simulink library "wt_blockset_v3"  (Simulink 6.0)
settings: Solver=ode45  SolverMode=SingleTasking  StartTime=0.0  StopTime=10.0  RelTol=1e-3
undefined symbols (not defined in the file): f1, get, j, Kmode, Type, u0
libraries: simulink_extras x12, simulink3 x5, simulink x4, dspinverses x1, dspmtrx3 x1, dspsnks4 x1
(part 2 of 7)

== system wt_blockset_v3/Electrical Machinery/Simulink Blocks  based Models ==
  note: Electric Machines Dynamic Models
  note: RMS Models
  note: Simulink Blocks
      |  based Models
  note: Special Models
  note: DQ Reference frame
  note: ABC/abc Models
  note: Salient Pole
      | Synchronous Machine
  note: Salient Pole
      | Synchronous Machine
  note: Reduced Order Models
  note: Permanent Magnet
      | Synchronous Machine
  note: Permanent Magnet
      | Synchronous Machine
  ABC/abc Squirell-Cage Induction Machine : Subsystem  mask(ABC/abc model of Squirrel Cage Induction Machine){Op_Mode=Generator, ConnType=Y, stator=[0.005 4.0744e-004], rotor=[0.0089 2.9921e-004], Lm=0.0160, p=2, init_cond=[0 0 0 0 0 0 0]}
      mask prompts: Op_Mode "Operating mode"; ConnType "Connection type"; stator "Stator windings [Rs Lsgm_s] [ohms H]"; rotor "Rotor windings [Rr Lsgm_r] [ohms H]"; Lm "Magnetizing inductance [H]"; p "Number of poles pair"; init_cond "Initial condition [iA iB iC ia ib ic theta]"
      mask help:
      | Implements an ABC/abc model for squirrel-cage induction machine.
      | Currents as state variable.
      mask init:
      | %%%%%%%%%%%%%%%%%%%%%%%%%%%%%%%%%%%%%%%%%%%%%%%%%%%%%%%%%%%%%%%%%%%%%%%%%%%%
      | % Matrix Coefficients for ABC/abc Model of Squirrel Cage Induction Machine %
      | %                       Last Update 10.05.20002                            %
      | %%%%%%%%%%%%%%%%%%%%%%%%%%%%%%%%%%%%%%%%%%%%%%%%%%%%%%%%%%%%%%%%%%%%%%%%%%%%
      | 
      | Rs=stator(1);
      | Lsgm_s=stator(2);
      | 
      | Rr=rotor(1);
      | Lsgm_r=rotor(2);
      | 
      | Msr=2*Lm/3;
      | 
      | %Self inductances
      | Ls=Lsgm_s+Lm;
      | Lr=Lsgm_r+Lm;
      | 
      | K1=Ls*Lr/(Msr^2);
      | 
      | K2=(K1-3/4)/(K1-9/4);
      | 
      | K3=-(3/4)/(K1-9/4);
      | 
      | K4=-(1/Msr)/(K1-9/4);
      | 
      | dlt=2*pi/3;
      | 
      | a11=K2*Rs/Ls;
      | a12=K3*Rs/Ls;
      | a13=3*Msr*sqrt(3)*K4/4;
      | a14=K4*Rr;
      | a15=Msr*(K2-K3)/Ls;
      | a16=K2/Ls;
      | a17=K3/Ls;
      | 
      | a31=K4*Rs;
      | a32=Msr*(K2-K3)/Lr;
      | a33=K2*Rr/Lr;
      | a34=K3*Rr/Lr;
      | a35=3*Msr*sqrt(3)*K4/4;
      | a36=K4;
      | if ConnType==1,Type=1;else Type=-1;end
      | if Op_Mode==1, Kmode=1;else Kmode=-1;end
      mask StyleString: popup(Motor|Generator),popup(Y|D),edit,edit,edit,edit,edit
      mask Display: disp('ABC/abc\nSC_IM')
  ABC/abc Wound Rotor Induction Machine : Subsystem  mask(ABC/abc model of Wound Rotor Induction Machine){stator=[0.005 4.0744e-004], rotor=[0.0089 2.9921e-004], Lm=0.0160, p=2, init_cond=[0 0 0 0 0 0 0]}
      mask prompts: stator "Stator windings [Rs Lsgm_s] [ohms H]"; rotor "Rotor windings [Rr Lsgm_r] [ohms H]"; Lm "Magnetizing inductance [H]"; p "Number of poles pair"; init_cond "Initial condition [iA iB iC ia ib ic theta]"
      mask help:
      | Implements an ABC/abc model for wound-rotor induction machine.
      | Currents as state variable.
      mask init:
      | %%%%%%%%%%%%%%%%%%%%%%%%%%%%%%%%%%%%%%%%%%%%%%%%%%%%%%%%%%%%%%%%%%%%%%%%%%%%
      | % Matrix Coefficients for ABC/abc Model of Wound Rotor Induction Machine %
      | %                       Last Update 10.05.20002                            %
      | %%%%%%%%%%%%%%%%%%%%%%%%%%%%%%%%%%%%%%%%%%%%%%%%%%%%%%%%%%%%%%%%%%%%%%%%%%%%
      | 
      | Rs=stator(1);
      | Lsgm_s=stator(2);
      | 
      | Rr=rotor(1);
      | Lsgm_r=rotor(2);
      | 
      | Msr=2*Lm/3;
      | 
      | %Self inductances
      | Ls=Lsgm_s+Lm;
      | Lr=Lsgm_r+Lm;
      | 
      | K1=Ls*Lr/(Msr^2);
      | 
      | K2=(K1-3/4)/(K1-9/4);
      | 
      | K3=-(3/4)/(K1-9/4);
      | 
      | K4=-(1/Msr)/(K1-9/4);
      | 
      | dlt=2*pi/3;
      | 
      | a11=K2*Rs/Ls;
      | a12=K3*Rs/Ls;
      | a13=3*Msr*sqrt(3)*K4/4;
      | a14=K4*Rr;
      | a15=Msr*(K2-K3)/Ls;
      | a16=K2/Ls;
      | a17=K3/Ls;
      | a18=K4;
      | 
      | a31=K4*Rs;
      | a32=Msr*(K2-K3)/Lr;
      | a33=K2*Rr/Lr;
      | a34=K3*Rr/Lr;
      | a35=3*Msr*sqrt(3)*K4/4;
      | a36=K4;
      | a37=K2/Lr;
      | a38=K3/Lr;
      mask Display: disp('ABC/abc\nWR_IM')
  Permanent Magnet Synchronous Machine with iron losses : Subsystem  mask{R=6.1, T=20, Ld=.043, Lq=.043, Ke=.165, p=2, s=Without iron losses}
      mask prompts: R "Rs [ohm] -stator resitance"; T "T [C] temperature of PMSM"; Ld "Ld [H] d-axis inductance"; Lq "Lq [H] - q-axis inductance"; Ke "Ke [Wb] - magnet flux"; p "p, pole pairs"; s "Iron Losses switch"
      mask init:
      | Rs=R*(1+.009*(T-20));
      mask StyleString: edit,edit,edit,edit,edit,edit,popup(With iron losses| Without iron losses)
      mask Display: disp('PM_SM')
  RMS Wound Rotor Induction Machine : Subsystem  mask(Complex Steady-State Induction Machine){rated_vi=[960 1310], rated_fp=[50 2], standstill=[8.8 79.5], stator=[0.005 4.074e-4], rotor=[0.0089 2.992e-4], Lm=16.0428e-3}
      mask prompts: rated_vi "Rated voltage / current per phase [Vph_r (V), Iph_r (A)]"; rated_fp "Base frequency,  Number of pole pairs [fs (Hz), p]"; standstill "Starting current,  Phase angle at standstill [Ist (pu), phi_st (deg)]"; stator "Stator parameters [Rs (ohms), Lsgm_s (H)]"; rotor "Rotor parameters [Rr (ohms), Lsgm_r (H)]"; Lm "Magnetizing inductance [H]"
      mask help:
      | Complex Steady-State Model of Induction Machine.
      | Deep-bar effect taken into account.
      mask init:
      | p=rated_fp(2); omg_synch=2*pi*rated_fp(1);
      | Xm=omg_synch*Lm;
      | Rs=stator(1); Xsgm_s= omg_synch*stator(2); Xs=Xsgm_s+Xm;
      | Rr=rotor(1); Xsgm_r=omg_synch*rotor(2); Xr=Xsgm_r+Xm;
      | sbd=Rr*sqrt((Rs^2+Xs^2)/((Xm^2-Xs*Xr)^2+(Rs*Xr)^2));
      | Rr_sc=(rated_vi(1)*sqrt(1/(1+(tan(standstill(2)*pi/180))^2))/standstill(1)/rated_vi(2)-Rs);
      | kr=Rr_sc/Rr;
      | kx=(tan(standstill(2)*pi/180)*(Rs+Rr_sc)-Xsgm_s)/Xsgm_r;
      mask Display: disp('Steady_State\nModel')
  RMS  Squirrel Cage Induction Machine : Subsystem  mask(Squirrel-Cage Induction Machine){rated_vi=[960 1310], rated_fp=[50 2], standstill=[8.8 79.5], stator=[0.005 0.128], rotor=[0.0089 0.094], Xm=5.04}
      mask prompts: rated_vi "Rated voltage / current per phase [Vph_r (V), Iph_r (A)]"; rated_fp "Base frequency,  Number of pole pairs [fs (Hz), p]"; standstill "Starting current,  Phase angle at standstill [Ist (pu), phi_st (deg)]"; stator "Stator parameters [Rs Xsgm_s]  [ohms]"; rotor "Rotor parameters [Rr Xsgm_r] [ohms]"; Xm "Magnetizing reactance [ohms]"
      mask help: Steady-State Model of Squirrel-cage Induction Machine
      mask init:
      | %%%%%%%%%%%%%%%%%%%%%%%%%%%%%%%%%%%%%%%%%%%%%%%%%%%%%%%%%%%%%%%%%%%%%%%%%%%%%%%%%%%%%
      | % Initialisation file for Squirrel-Cage Induction Machine with Deep Bar Effect      %
      | % RMS model
      | %                           Last Update 06.06.2002 by FI                             %
      | %%%%%%%%%%%%%%%%%%%%%%%%%%%%%%%%%%%%%%%%%%%%%%%%%%%%%%%%%%%%%%%%%%%%%%%%%%%%%%%%%%%%%
      | 
      | %base angular speed
      | omg_base=2*pi*rated_fp(1);
      | 
      | %%%%%%%%%%%%%%%%%%%%%%%%%%%%
      | %Stator winding
      | %%%%%%%%%%%%%%%%%%%%%%%%%%%%
      | 
      | %Stator resistance
      | Rs=stator(1);
      | 
      | %Stator leakage inductance
      | Xsgm_s= stator(2);
      | 
      | %Stator self-inductance
      | Xs=Xsgm_s+Xm;
      | 
      | %%%%%%%%%%%%%%%%%%%%%%%%%%%%
      | %Rotor winding
      | %%%%%%%%%%%%%%%%%%%%%%%%%%%%
      | 
      | %Rotor resistance for rated operating point
      | Rr=rotor(1); 
      | 
      | %Rotor leakage inductance for rated operating point
      | Xsgm_r=rotor(2);
      | 
      | %Rotor self-inductance
      | Xr=Xsgm_r+Xm;
      | 
      | %Number of pole pairs
      | p=rated_fp(2);
      | 
      | %Breakdown slip
      | sbd=Rr*sqrt((Rs^2+Xs^2)/((Xm^2-Xs*Xr)^2+(Rs*Xr)^2));
      | 
      | %rotor resistance at start_up
      | Rr_sc=(rated_vi(1)*sqrt(1/(1+(tan(standstill(2)*pi/180))^2))/standstill(1)/rated_vi(2)-Rs);
      | 
      | %rotor resistance displacement factor
      | kr=Rr_sc/Rr;
      | 
      | %rotor reactance displacement factor
      | kx=(tan(standstill(2)*pi/180)*(Rs+Rr_sc)-Xsgm_s)/Xsgm_r;
      mask Display: disp('Steady_State\nModel')
  Reduced Order Model Induction Machine : Subsystem  mask(Generalized 3rd order model of Asynchronous Generator){stator=[0.0011, 7e-005], rotor=[0.0013, 7.5e-005], magnetization=2.9936e-003, rated_fp=[50 2], init_cond=[0 0]}
      mask prompts: stator "Stator parameters [Rs (ohms), Lsgm_s (H)]"; rotor "Rotor parameters [Rr (ohms), Lsgm_r (H)]"; magnetization "Magnetizing inductance Lm (H)"; rated_fp "Base frequency, Number of pole pairs [fs (Hz), p]"; init_cond "Initial conditions [fi_dr (Wb), fi_qr(Wb)]"
      mask help: Implements a generalized 3rd order model for Asynchronous Generator in synchronous reference frame.
      mask init:
      | Rs=stator(1);Lsgm_s=stator(2);
      | Rr=rotor(1);Lsgm_r=rotor(2);Lm=magnetization;
      | omg_e=2*pi*rated_fp(1);p=rated_fp(2);
      | Lss=Lsgm_s+Lm;Lrr=Lsgm_r+Lm;D=Lss*Lrr-Lm^2;
      | tau_sr=Rs*Lrr/D;tau_rm=Rr*Lm/D;sigma_r=Lm/Lrr;sigma_s=Lm/Lss;
      | alpha=1/(1+(omg_e/tau_sr)^2);
      | M=[Lss 0 Lm 0;0 Lss 0 Lm;Lm 0 Lrr 0;0 Lm 0 Lrr];
      | Q=inv(M);
      mask Display: disp('IM\n3rd Order Model')
  Salient-Pole Synchronous Machine constant parameters : Subsystem  mask{stator_winding=[2.34e-3 3.92e-4], field_winding=[5e-4 6.69246e-4], rotor_winding=[17.36e-3 5.22558e-4 16.75e-3 3.36082e-4], mag_ind=[2.3844e-3 1.1759e-3], p=32}
      mask prompts: stator_winding "Stator winding [Rs Lsgm_s]"; field_winding "Field winding [Rf Lsgm_f]"; rotor_winding "Rotor winding [Rrd Lsgm_rd Rrq Lsgm_rq]"; mag_ind "Magnetizing inductances [Lmd Lmq]"; p "Number of pole pairs"
      mask init:
      | %%%%%%%%%%%%%%%%%%%%%%%%%%%%%%%%%%%%%%%%%%%%%%%%%%%%%%%%%%%%%%%%%%%%%%%%
      | % Matrix coefficients for DQ model of Salient-Pole Synchronous Machine %
      | %                   Last Update 10.05.2002                             %
      | %%%%%%%%%%%%%%%%%%%%%%%%%%%%%%%%%%%%%%%%%%%%%%%%%%%%%%%%%%%%%%%%%%%%%%%%
      | 
      | %Stator winding
      | Rs=stator_winding(1); Lsgm_s=stator_winding(2);
      | 
      | %Field winding
      | Rf=field_winding(1); Lsgm_f=field_winding(2);
      | 
      | %Rotor winding D axis
      | Rrd=rotor_winding(1); Lsgm_rd=rotor_winding(2);
      | 
      | %Rotor windin Q axis
      | Rrq=rotor_winding(3); Lsgm_rq=rotor_winding(4);
      | 
      | %Magnetizing inductances DQ axis
      | Lmd=mag_ind(1); Lmq=mag_ind(2);
      | 
      | %Self Inductances
      | Lssd=Lsgm_s+Lmd;
      | Lssq=Lsgm_s+Lmq;
      | Lsf=Lsgm_f+Lmd;
      | Lsrd=Lsgm_rd+Lmd;
      | Lsrq=Lsgm_rq+Lmq;
      | 
      | %Coeffients
      | Ksgm_d=Lsgm_s*Lsgm_f*Lsgm_rd+Lmd*(Lsgm_s*Lsgm_f+Lsgm_f*Lsgm_rd+Lsgm_rd*Lsgm_s);
      | Ksgm_q=Lsgm_s*Lsgm_rq+Lmq*(Lsgm_s+Lsgm_rq);
      | 
      | Ksgm_frd=Lsgm_f*Lsgm_rd+Lmd*(Lsgm_f+Lsgm_rd);
      | Ksgm_srd=Lsgm_s*Lsgm_rd+Lmd*(Lsgm_s+Lsgm_rd);
      | Ksgm_sf=Lsgm_f*Lsgm_s+Lmd*(Lsgm_f+Lsgm_s);
      | 
      | %Matrix coefficients
      | a11=-Rs*Ksgm_frd/Ksgm_d;
      | a12=Lssq*Ksgm_frd/Ksgm_d;
      | a13=Rf*Lsgm_rd*Lmd/Ksgm_d;
      | a14=Rrd*Lsgm_f*Lmd/Ksgm_d;
      | a15=Lmq*Ksgm_frd/Ksgm_d;
      | a16=Ksgm_frd/Ksgm_d;
      | a17=-Lsgm_rd*Lmd/Ksgm_d;
      | 
      | a21=-Lssd*Lsrq/Ksgm_q;
      | a22=-Rs*Lsrq/Ksgm_q;
      | a23=-Lsrq*Lmd/Ksgm_q;
      | a24=-Lsrq*Lmd/Ksgm_q;
      | a25=Rrq*Lmq/Ksgm_q;
      | a26=Lsrq/Ksgm_q;
      | 
      | a31=+Rs*Lsgm_rd*Lmd/Ksgm_d;
      | a32=-Lssq*Lsgm_rd*Lmd/Ksgm_d;
      | a33=-Rf*Ksgm_srd/Ksgm_d;
      | a34=Rrd*Lsgm_s*Lmd/Ksgm_d;
      | a35=-Lsgm_rd*Lmd*Lmq/Ksgm_d;
      | a36=-Lsgm_rd*Lmd/Ksgm_d;
      | a37=Ksgm_srd/Ksgm_d;
      | 
      | a41=Rs*Lsgm_f*Lmd/Ksgm_d;
      | a42=-Lsgm_f*Lssq*Lmd/Ksgm_d;
      | a43=Rf*Lsgm_s*Lmd/Ksgm_d;
      | a44=-Rrd*Ksgm_sf/Ksgm_d;
      | a45=-Lsgm_f*Lmd*Lmq/Ksgm_d;
      | a46=-Lsgm_f*Lmd/Ksgm_d;
      | a47=-Lsgm_s*Lmd/Ksgm_d;
      | 
      | a51=Lssd*Lmq/Ksgm_q;
      | a52=Rs*Lmq/Ksgm_q;
      | a53=Lmd*Lmq/Ksgm_q;
      | a54=Lmd*Lmq/Ksgm_q;
      | a55=-Rrq*Lssq/Ksgm_q;
      | a56=-Lmq/Ksgm_q;
      mask Display: disp('SP_SM')
  Squirrel Cage Induction Machine constant parameters : Subsystem  mask(Squirrel-Cage Induction Machine){Op_Mode=Generator, ConnType=Y, stator=[3.67 9.2e-3], rotor=[2.32 12.29e-3], Lm=0.235, p=2, x0=[0 0 0 0 0]}
      mask prompts: Op_Mode "Operating mode"; ConnType "Connection type"; stator "Stator parameters [Rs (ohm), Lsgm_s(H)]"; rotor "Rotor parameters [Rr (ohm) Lsgm_r (H)]"; Lm "Mutual inductance [H]"; p "Number of pole pairs"; x0 "Initial conditions [ids iqs idr iqr theta]"
      mask help:
      | Implements a dq model in rotor reference frame for squirrel-cage induction machine.
      | Currents as state variable.
      mask init:
      | if ConnType==1,Type=1;else Type=-1;end
      | if Op_Mode==1, Kmode=1;else Kmode=-1;end
      | Rs=stator(1); Lsgms= stator(2); Lss=Lsgms+Lm;
      | Rr=rotor(1); Lsgmr=rotor(2); Lsr=Lsgmr+Lm;
      | sigma=1-(Lm*Lm)/(Lss*Lsr);
      mask StyleString: popup(Motor|Generator),popup(Y|D),edit,edit,edit,edit,edit
      mask Display: disp('SC_IM')
  Squirrel Cage  Induction Machine  with Deep Bar Effect : Subsystem  mask(Squirrel-Cage Induction Machine with Deep Bar Effect){Op_Mode=Motor, ConnType=Y, rated_vi=[960 1310], rated_fp=[50 2], standstill=[8.8 79.5], stator=[0.005 4.074e-4], rotor=[0.0089 2.992e-4], Lm=16.0428e-3, x0=[0 0 0 0 0]}
      mask prompts: Op_Mode "Operating mode"; ConnType "Connection type"; rated_vi "Rated voltage / current per-phase [Vph_r (V), Iph_r (A)]"; rated_fp "Base frequency,  Number of pole pairs [fs (Hz), p]"; standstill "Starting current,  Phase angle at standstill [Ist (pu), phi_st (deg)]"; stator "Stator [Rs (ohm), Lsgm_s (H)]"; rotor "Rotor [Rr (ohm), Lsgm_r (H)]"; Lm "Magnetizing inductance Lm [H]"; x0 "Initial conditions [ids iqs idr iqr theta]"
      mask help: Implement a DQ Model in rotor reference frame for Squirrel-Cage Induction Machine with Deep bar effect
      mask init:
      | if ConnType==1,Type=1;else Type=-1;end
      | if Op_Mode==1, Kmode=1;else Kmode=-1;end
      | %%%%%%%%%%%%%%%%%%%%%%%%%%%%%%%%%%%%%%%%%%%%%%%%%%%%%%%%%%%%%%%%%%%%%%%%%%%%%%%%%%%%%
      | % Initialisation file for squirrel-Cage Induction Machine with Deep Bar Effect      %
      | %                          Last Update 15.05.2002 by FI                             %
      | %%%%%%%%%%%%%%%%%%%%%%%%%%%%%%%%%%%%%%%%%%%%%%%%%%%%%%%%%%%%%%%%%%%%%%%%%%%%%%%%%%%%%
      | 
      | %base angular speed
      | omg_base=2*pi*rated_fp(1);
      | 
      | %Magnetizing reactance
      | Xm=omg_base*Lm;
      | %%%%%%%%%%%%%%%%%%%%%%%%%%%%
      | %Stator winding
      | %%%%%%%%%%%%%%%%%%%%%%%%%%%%
      | 
      | %Stator resistance
      | Rs=stator(1);
      | 
      | %Stator leakage inductance
      | Lsgms= stator(2);
      | Xsgm_s=omg_base*Lsgms;
      | 
      | %Stator self-inductance
      | Lss=Lsgms+Lm;
      | Xs=omg_base*Lss;
      | 
      | %%%%%%%%%%%%%%%%%%%%%%%%%%%%
      | %Rotor winding
      | %%%%%%%%%%%%%%%%%%%%%%%%%%%%
      | 
      | %Rotor resistance for rated operating point
      | Rr=rotor(1); 
      | 
      | %Rotor leakage inductance for rated operating point
      | Lsgmr=rotor(2);
      | Xsgm_r=omg_base*rotor(2);
      | 
      | %Rotor self-inductance
      | Lsr=rotor(2)+Lm;
      | Xr=omg_base*Lsr;
      | 
      | %Number of pole pairs
      | p=rated_fp(2);
      | 
      | %Breakdown slip
      | sbd=Rr*sqrt((Rs^2+Xs^2)/((Xm^2-Xs*Xr)^2+(Rs*Xr)^2));
      | 
      | %rotor resistance at start_up
      | Rr_sc=(rated_vi(1)*sqrt(1/(1+(tan(standstill(2)*pi/180))^2))/standstill(1)/rated_vi(2)-Rs);
      | 
      | %rotor resistance displacement factor
      | kr=Rr_sc/Rr;
      | 
      | %rotor reactance displacement factor
      | kx=(tan(standstill(2)*pi/180)*(Rs+Rr_sc)-Xsgm_s)/Xsgm_r;
      mask StyleString: popup(Motor|Generator),popup(Y|D),edit,edit,edit,edit,edit,edit,edit
      mask Display: disp('SC_IM')
  Wound Rotor Induction Machine constant parameters : Subsystem  mask(3-phase Wound Rotor Induction Machine){stator=[0.01 95.5e-6], rotor=[0.01 95.5e-6], Lm=0.0955, p=2, x0=[0 0 0 0 0]}
      mask prompts: stator "Stator parameters [Rs (ohm), Lsgm_s (H)]"; rotor "Rotor parameters [Rr (ohm), Lsgm_r (H)]"; Lm "Magnetizing inductance [H]"; p "Number of poles pair"; x0 "Initial conditions [ids iqs idr' iqr' theta]"
      mask init:
      | Rs=stator(1); Lsgm_s=stator(2);
      | Rr=rotor(1); Lsgm_r=rotor(2);
      | Lss=Lsgm_s+Lm;
      | Lsr=Lsgm_r+Lm;
      | sigma=1-(Lm*Lm)/(Lss*Lsr);
      mask Display: disp('WR_IM')
  "Wound Rotor Induction Machine with Deep Bar Effect " : Subsystem  mask(3-phase Wound Rotor Induction Machine){rated_vi=[960 1310], rated_fp=[50 2], standstill=[8.8 79.5], stator=[0.005 4.074e-4], rotor=[0.0089 2.992e-4], Lm=16.0428e-3, x0=[0 0 0 0 0]}
      mask prompts: rated_vi "Rated voltage / current per-phase [Vph_r (V), Iph_r (A)]"; rated_fp "Base frequency,  Number of pole pairs [fs (Hz), p]"; standstill "Starting current,  Phase angle at standstill [Ist (pu), phi_st (deg)]"; stator "Stator [Rs (ohm), Lsgm_s (H)]"; rotor "Rotor [Rr (ohm), Lsgm_r (H)]"; Lm "Magnetizing inductance Lm [H]"; x0 "Initial conditions [ids iqs idr' iqr' theta]"
      mask init:
      | %%%%%%%%%%%%%%%%%%%%%%%%%%%%%%%%%%%%%%%%%%%%%%%%%%%%%%%%%%%%%%%%%%%%%%%%%%%%%%%%%%%%%
      | % Initialisation file for Wound Rotor Induction Machine with Deep Bar Effect      %
      | %                          Last Update 24.09.2004 by FI                             %
      | %%%%%%%%%%%%%%%%%%%%%%%%%%%%%%%%%%%%%%%%%%%%%%%%%%%%%%%%%%%%%%%%%%%%%%%%%%%%%%%%%%%%%
      | 
      | %base angular speed
      | omg_base=2*pi*rated_fp(1);
      | 
      | %Magnetizing reactance
      | Xm=omg_base*Lm;
      | %%%%%%%%%%%%%%%%%%%%%%%%%%%%
      | %Stator winding
      | %%%%%%%%%%%%%%%%%%%%%%%%%%%%
      | 
      | %Stator resistance
      | Rs=stator(1);
      | 
      | %Stator leakage inductance
      | Lsgms= stator(2);
      | Xsgm_s=omg_base*Lsgms;
      | 
      | %Stator self-inductance
      | Lss=Lsgms+Lm;
      | Xs=omg_base*Lss;
      | 
      | %%%%%%%%%%%%%%%%%%%%%%%%%%%%
      | %Rotor winding
      | %%%%%%%%%%%%%%%%%%%%%%%%%%%%
      | 
      | %Rotor resistance for rated operating point
      | Rr=rotor(1); 
      | 
      | %Rotor leakage inductance for rated operating point
      | Lsgmr=rotor(2);
      | Xsgm_r=omg_base*rotor(2);
      | 
      | %Rotor self-inductance
      | Lsr=rotor(2)+Lm;
      | Xr=omg_base*Lsr;
      | 
      | %Number of pole pairs
      | p=rated_fp(2);
      | 
      | %Breakdown slip
      | sbd=Rr*sqrt((Rs^2+Xs^2)/((Xm^2-Xs*Xr)^2+(Rs*Xr)^2));
      | 
      | %rotor resistance at start_up
      | Rr_sc=(rated_vi(1)*sqrt(1/(1+(tan(standstill(2)*pi/180))^2))/standstill(1)/rated_vi(2)-Rs);
      | 
      | %rotor resistance displacement factor
      | kr=Rr_sc/Rr;
      | 
      | %rotor reactance displacement factor
      | kx=(tan(standstill(2)*pi/180)*(Rs+Rr_sc)-Xsgm_s)/Xsgm_r;
      mask Display: disp('WR_IM')

== system wt_blockset_v3/Grid Models/3-ph line 1 ==
  note: VfR
  note: VbR
  note: VfS
  note: VbS
  iS_abc : Inport  Port=1  LatchInput=off
  iR_abc : Inport  Orientation=left  Port=2  LatchInput=off
  1 : Gain  Gain=atten  SaturateOnIntegerOverflow=on
  2 : Gain  Orientation=left  Gain=atten  SaturateOnIntegerOverflow=on
  Gain1 : Gain  Orientation=left  Gain=2  SaturateOnIntegerOverflow=on
  Gain6 : Gain  Gain=2  SaturateOnIntegerOverflow=on
  R_to_S delay : TransportDelay  Orientation=left  DelayTime=tdelay  BufferSize=buffer_size
  S_to_R delay : TransportDelay  DelayTime=tdelay  BufferSize=buffer_size
  Sum1 : Sum  Orientation=up  SaturateOnIntegerOverflow=on  InputSameDT=on
  Sum2 : Sum  Inputs=+-  SaturateOnIntegerOverflow=on  InputSameDT=on
  Sum4 : Sum  Orientation=down  Inputs=+-  SaturateOnIntegerOverflow=on  InputSameDT=on
  Sum5 : Sum  Orientation=left  Inputs=-+  SaturateOnIntegerOverflow=on  InputSameDT=on
  Zc1 : Gain  Orientation=up  Gain=Zc  SaturateOnIntegerOverflow=on
  Zc2 : Gain  Orientation=down  Gain=Zc  SaturateOnIntegerOverflow=on
  VS_abc : Outport  Orientation=left  InitialOutput=0
  "VR_abc " : Outport  Port=2  InitialOutput=0
  wires:
  1/1 -> Sum5/1, Gain6/1
  Sum1/1 -> Sum2/1, VS_abc/1
  iR_abc/1 -> Zc2/1
  iS_abc/1 -> Zc1/1
  Sum4/1 -> "VR_abc "/1, Sum5/2
  Sum5/1 -> R_to_S delay/1
  Zc2/1 -> Sum4/2
  Sum2/1 -> S_to_R delay/1
  Zc1/1 -> Sum1/1
  Gain6/1 -> Sum4/1
  Gain1/1 -> Sum1/2
  S_to_R delay/1 -> 1/1
  R_to_S delay/1 -> 2/1
  2/1 -> Gain1/1, Sum2/2

== system wt_blockset_v3/Grid Models/3-ph line 2 ==
  note: VbS
  note: VfS
  note: VbR
  note: VfR
  VS_abc : Inport  Port=1  LatchInput=off
  iR_abc : Inport  Orientation=left  Port=2  LatchInput=off
  3 : Gain  Gain=atten  SaturateOnIntegerOverflow=on
  4 : Gain  Orientation=left  Gain=atten  SaturateOnIntegerOverflow=on
  Gain3 : Gain  Gain=2  SaturateOnIntegerOverflow=on
  Gain4 : Gain  Orientation=left  Gain=2  SaturateOnIntegerOverflow=on
  R_to_S delay1 : TransportDelay  Orientation=left  DelayTime=tdelay  BufferSize=buffer_size
  S_to_R delay1 : TransportDelay  DelayTime=tdelay  BufferSize=buffer_size
  Sum2 : Sum  Inputs=+-  SaturateOnIntegerOverflow=on  InputSameDT=on
  Sum3 : Sum  Inputs=+-  SaturateOnIntegerOverflow=on  InputSameDT=on
  Sum6 : Sum  Orientation=down  Inputs=+-  SaturateOnIntegerOverflow=on  InputSameDT=on
  Sum7 : Sum  Orientation=left  Inputs=-+  SaturateOnIntegerOverflow=on  InputSameDT=on
  Zc3 : Gain  Gain=1/Zc  SaturateOnIntegerOverflow=on
  Zc4 : Gain  Orientation=down  Gain=Zc  SaturateOnIntegerOverflow=on
  break algebraic loop1 : Subsystem  mask(Transfer function){K=1, T=1e-5, x0=445}
      mask prompts: K "Gain"; T "Time constant"; x0 "Initial condition"
      mask help: Implements a transfer function K/(sT+1) with initial condition.
  iS_abc : Outport  InitialOutput=0
  "VR_abc " : Outport  Port=2  InitialOutput=0
  wires:
  4/1 -> Sum3/2, Gain4/1
  R_to_S delay1/1 -> 4/1
  S_to_R delay1/1 -> 3/1
  Gain3/1 -> Sum6/1
  Sum3/1 -> S_to_R delay1/1
  Zc4/1 -> Sum6/2
  Sum7/1 -> R_to_S delay1/1
  Sum6/1 -> Sum7/2, "VR_abc "/1
  3/1 -> Sum7/1, Gain3/1
  VS_abc/1 -> Sum2/1, Sum3/1
  iR_abc/1 -> Zc4/1
  Zc3/1 -> break algebraic loop1/1(In1)
  Sum2/1 -> Zc3/1
  Gain4/1 -> Sum2/2
  break algebraic loop1/1(Out1) -> iS_abc/1

== system wt_blockset_v3/Grid Models/3-phase 3 limb  C S-Function ==
  v_UVW : Inport  Port=1  LatchInput=off
  i_uvw : Inport  Port=2  LatchInput=off
  Mux : Mux  Inputs=2
  Ropen : Gain  Orientation=down  Gain=1000000  SaturateOnIntegerOverflow=on
  Ropen1 : Gain  Gain=-sqrt(3)  SaturateOnIntegerOverflow=on
  S-Function : S-Function  FunctionName=trafo3limb_abc_zcs  Parameters=a b init_cond
  Selector iABC : Selector  Elements=[1 2 3]  InputPortWidth=6
  Selector iabc : Selector  Elements=[4 5 6]  InputPortWidth=6
  Sum : Sum  Inputs=|+-  SaturateOnIntegerOverflow=on  InputSameDT=on
  phase->line2 : Subsystem
  turns ratio : Gain  Gain=-alpha_T  SaturateOnIntegerOverflow=on
  turns ratio1 : Gain  Gain=alpha_T  SaturateOnIntegerOverflow=on
  i_UVW : Outport
  v_uvw : Outport  Port=2
  wires:
  i_uvw/1 -> Sum/2
  turns ratio1/1 -> Sum/1
  Ropen1/1 -> v_uvw/1
  Ropen/1 -> turns ratio/1, Ropen1/1
  Sum/1 -> Ropen/1
  S-Function/1 -> Selector iabc/1, Selector iABC/1
  Mux/1 -> S-Function/1
  turns ratio/1 -> Mux/2
  v_UVW/1 -> Mux/1
  phase->line2/1(out) -> i_UVW/1
  Selector iABC/1 -> phase->line2/1(in)
  Selector iabc/1 -> turns ratio1/1

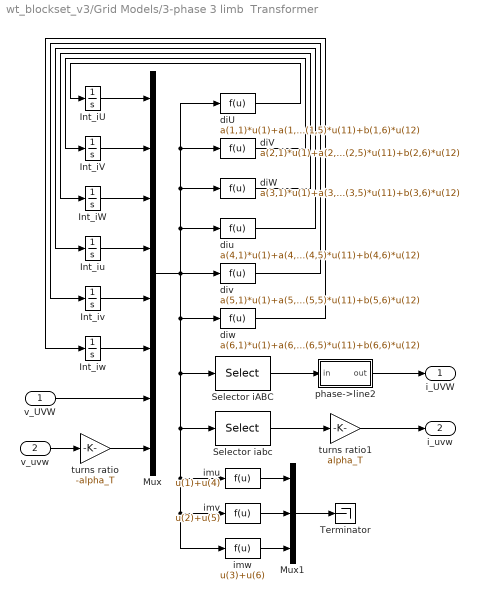
== system wt_blockset_v3/Grid Models/3-phase 3 limb  Transformer ==
  v_UVW : Inport  Port=1  LatchInput=off
  v_uvw : Inport  Port=2  LatchInput=off
  Int_iU : Integrator
  Int_iV : Integrator
  Int_iW : Integrator
  Int_iu : Integrator
  Int_iv : Integrator
  Int_iw : Integrator
  Mux : Mux  Inputs=[1 1 1 1 1 1 3 3]
  Mux1 : Mux  Inputs=3
  Selector iABC : Selector  Elements=[1 2 3]  InputPortWidth=12
  Selector iabc : Selector  Elements=[4 5 6]  InputPortWidth=12
  Terminator : Terminator
  diU : Fcn  Expr=a(1,1)*u(1)+a(1,2)*u(2)+a(1,3)*u(3)+a(1,4)*u(4)+a(1,5)*u(5)+a(1,6)*u(6)+b(1,1)*u(7)+b(1,2)*u(8)+b(1,3)*u(9)+b(1,4)*u(10)+b(1,5)*u(11)+b(1,6)*u(12)
  diV : Fcn  Expr=a(2,1)*u(1)+a(2,2)*u(2)+a(2,3)*u(3)+a(2,4)*u(4)+a(2,5)*u(5)+a(2,6)*u(6)+b(2,1)*u(7)+b(2,2)*u(8)+b(2,3)*u(9)+b(2,4)*u(10)+b(2,5)*u(11)+b(2,6)*u(12)
  diW : Fcn  Expr=a(3,1)*u(1)+a(3,2)*u(2)+a(3,3)*u(3)+a(3,4)*u(4)+a(3,5)*u(5)+a(3,6)*u(6)+b(3,1)*u(7)+b(3,2)*u(8)+b(3,3)*u(9)+b(3,4)*u(10)+b(3,5)*u(11)+b(3,6)*u(12)
  diu : Fcn  Expr=a(4,1)*u(1)+a(4,2)*u(2)+a(4,3)*u(3)+a(4,4)*u(4)+a(4,5)*u(5)+a(4,6)*u(6)+b(4,1)*u(7)+b(4,2)*u(8)+b(4,3)*u(9)+b(4,4)*u(10)+b(4,5)*u(11)+b(4,6)*u(12)
  div : Fcn  Expr=a(5,1)*u(1)+a(5,2)*u(2)+a(5,3)*u(3)+a(5,4)*u(4)+a(5,5)*u(5)+a(5,6)*u(6)+b(5,1)*u(7)+b(5,2)*u(8)+b(5,3)*u(9)+b(5,4)*u(10)+b(5,5)*u(11)+b(5,6)*u(12)
  diw : Fcn  Expr=a(6,1)*u(1)+a(6,2)*u(2)+a(6,3)*u(3)+a(6,4)*u(4)+a(6,5)*u(5)+a(6,6)*u(6)+b(6,1)*u(7)+b(6,2)*u(8)+b(6,3)*u(9)+b(6,4)*u(10)+b(6,5)*u(11)+b(6,6)*u(12)
  imu : Fcn  Expr=u(1)+u(4)
  imv : Fcn  Expr=u(2)+u(5)
  imw : Fcn  Expr=u(3)+u(6)
  phase->line2 : Subsystem
  turns ratio : Gain  Gain=-alpha_T  SaturateOnIntegerOverflow=on
  turns ratio1 : Gain  Gain=alpha_T  SaturateOnIntegerOverflow=on
  i_UVW : Outport
  i_uvw : Outport  Port=2
  wires:
  turns ratio/1 -> Mux/8
  Selector iabc/1 -> turns ratio1/1
  Selector iABC/1 -> phase->line2/1(in)
  v_uvw/1 -> turns ratio/1
  v_UVW/1 -> Mux/7
  diw/1 -> Int_iw/1
  div/1 -> Int_iv/1
  diu/1 -> Int_iu/1
  diW/1 -> Int_iW/1
  diV/1 -> Int_iV/1
  diU/1 -> Int_iU/1
  Int_iw/1 -> Mux/6
  Int_iv/1 -> Mux/5
  Int_iu/1 -> Mux/4
  Int_iW/1 -> Mux/3
  Int_iV/1 -> Mux/2
  Int_iU/1 -> Mux/1
  Mux/1 -> Selector iABC/1, Selector iabc/1, imu/1, imv/1, imw/1, diw/1, div/1, diU/1, diV/1, diW/1, diu/1
  turns ratio1/1 -> i_uvw/1
  phase->line2/1(out) -> i_UVW/1
  imu/1 -> Mux1/1
  imv/1 -> Mux1/2
  imw/1 -> Mux1/3
  Mux1/1 -> Terminator/1

== system wt_blockset_v3/Grid Models/3-phase source ==
  Mux3 : Mux  Inputs=3
  ua : Sin  Amplitude=sqrt(2)*Uf  Frequency=2*pi*fs  SampleTime=0
  ub : Sin  Amplitude=sqrt(2)*Uf  Frequency=2*pi*fs  Phase=-2*pi/3  SampleTime=0
  uc : Sin  Amplitude=sqrt(2)*Uf  Frequency=2*pi*fs  Phase=2*pi/3  SampleTime=0
  uRST : Outport  InitialOutput=0
  wires:
  uc/1 -> Mux3/3
  ub/1 -> Mux3/2
  Mux3/1 -> uRST/1
  ua/1 -> Mux3/1

== system wt_blockset_v3/Grid Models/Capacitor Bank RC ==
  V_RST : Inport  Port=1  LatchInput=off
  k : Inport  Port=2  LatchInput=off
  Branch A : TransferFcn  Numerator=[C 0]  Denominator=[R*C 1]
  Branch B : TransferFcn  Numerator=[C 0]  Denominator=[R*C 1]
  Branch C : TransferFcn  Numerator=[C 0]  Denominator=[R*C 1]
  Demux : Demux  Outputs=3
  Mux : Mux  Inputs=3
  Product : Product  SaturateOnIntegerOverflow=on  InputSameDT=on
  I_RST : Outport
  wires:
  k/1 -> Product/2
  Product/1 -> I_RST/1
  V_RST/1 -> Demux/1
  Mux/1 -> Product/1
  Branch C/1 -> Mux/3
  Branch B/1 -> Mux/2
  Branch A/1 -> Mux/1
  Demux/3 -> Branch C/1
  Demux/2 -> Branch B/1
  Demux/1 -> Branch A/1

== system wt_blockset_v3/Grid Models/Capacitor Bank RC modified ==
  V_RST : Inport  Port=1  LatchInput=off
  k : Inport  Port=2  LatchInput=off
  Branch A : TransferFcn  Numerator=[C 0]  Denominator=[R*C 1]
  Branch B : TransferFcn  Numerator=[C 0]  Denominator=[R*C 1]
  Branch C : TransferFcn  Numerator=[C 0]  Denominator=[R*C 1]
  Demux : Demux  Outputs=3
  Mux : Mux  Inputs=3
  Product : Product  SaturateOnIntegerOverflow=on  InputSameDT=on
  I_RST : Outport
  wires:
  k/1 -> Product/2
  Product/1 -> I_RST/1
  V_RST/1 -> Demux/1
  Mux/1 -> Product/1
  Branch C/1 -> Mux/3
  Branch B/1 -> Mux/2
  Branch A/1 -> Mux/1
  Demux/3 -> Branch C/1
  Demux/2 -> Branch B/1
  Demux/1 -> Branch A/1

== system wt_blockset_v3/Grid Models/Capacitor Bank RLC ==
  v_RST : Inport  Port=1  LatchInput=off
  k : Inport  Port=2  LatchInput=off
  Demux : Demux  Outputs=3
  Mux : Mux  Inputs=3
  Product : Product  SaturateOnIntegerOverflow=on  InputSameDT=on
  Transfer Fcn : TransferFcn  Numerator=[C 0]  Denominator=[L*C R*C 1]
  Transfer Fcn1 : TransferFcn  Numerator=[C 0]  Denominator=[L*C R*C 1]
  Transfer Fcn2 : TransferFcn  Numerator=[C 0]  Denominator=[L*C R*C 1]
  I_RST : Outport
  wires:
  v_RST/1 -> Demux/1
  Transfer Fcn2/1 -> Mux/3
  Transfer Fcn1/1 -> Mux/2
  Transfer Fcn/1 -> Mux/1
  Demux/1 -> Transfer Fcn/1
  Demux/2 -> Transfer Fcn1/1
  Demux/3 -> Transfer Fcn2/1
  k/1 -> Product/2
  Product/1 -> I_RST/1
  Mux/1 -> Product/1

== system wt_blockset_v3/Grid Models/Circuit breaker ==
  Vin_ABC : Inport  Orientation=left  Port=1  LatchInput=off
  Is_ABC : Inport  Orientation=left  Port=2  LatchInput=off
  CB : Inport  Orientation=left  Port=3  LatchInput=off
  Circuit breaker1 : Subsystem  Orientation=left
  Circuit breaker2 : Subsystem  Orientation=left
  Circuit breaker3 : Subsystem  Orientation=left
  Demux : Demux  Orientation=left  Outputs=3
  Demux1 : Demux  Orientation=left  Outputs=3
  Mux : Mux  Orientation=left  Inputs=3
  Vb_ABC : Outport  Orientation=left
  wires:
  Mux/1 -> Vb_ABC/1
  Circuit breaker3/1(vc) -> Mux/3
  Circuit breaker1/1(va) -> Mux/1
  Circuit breaker2/1(vb) -> Mux/2
  CB/1 -> Circuit breaker3/3(on/off), Circuit breaker2/3(on/off), Circuit breaker1/3(on/off)
  Demux1/3 -> Circuit breaker3/2(iT)
  Demux1/2 -> Circuit breaker2/2(iR)
  Demux1/1 -> Circuit breaker1/2(iS)
  Is_ABC/1 -> Demux1/1
  Demux/3 -> Circuit breaker3/1(Vin)
  Demux/1 -> Circuit breaker1/1(Vin)
  Vin_ABC/1 -> Demux/1
  Demux/2 -> Circuit breaker2/1(Vin)

== system wt_blockset_v3/Grid Models/DC-link circuit ==
  idc_inv : Inport  Port=1  LatchInput=off
  idc_red : Inport  Port=2  LatchInput=off
  Integrator : Integrator  InitialConditionSource=external
  Resistance : Gain  Gain=R  SaturateOnIntegerOverflow=on
  Sum : Sum  Inputs=|+-  SaturateOnIntegerOverflow=on  InputSameDT=on
  Sum1 : Sum  Inputs=|++  SaturateOnIntegerOverflow=on  InputSameDT=on
  capacitor : Gain  Gain=1/C  SaturateOnIntegerOverflow=on
  init_cond : Constant  Value=init_cond
  vdc : Outport
  wires:
  Sum1/1 -> vdc/1
  Sum/1 -> Resistance/1, capacitor/1
  idc_inv/1 -> Sum/2
  idc_red/1 -> Sum/1
  Resistance/1 -> Sum1/1
  capacitor/1 -> Integrator/1
  Integrator/1 -> Sum1/2
  init_cond/1 -> Integrator/2

== system wt_blockset_v3/Grid Models/GRID 1 ==
  uRST : Inport  Port=1  LatchInput=off
  Gain : Gain  Gain=X/(2*pi*fs)  SaturateOnIntegerOverflow=on
  Gain1 : Gain  Orientation=left  Gain=R  SaturateOnIntegerOverflow=on
  Integrator : Integrator
  Mux3 : Mux  Inputs=3
  Sum : Sum  Inputs=-+-  SaturateOnIntegerOverflow=on  InputSameDT=on
  ua : Sin  Amplitude=sqrt(2)*Uf  Frequency=2*pi*fs  SampleTime=0
  ub : Sin  Amplitude=sqrt(2)*Uf  Frequency=2*pi*fs  Phase=-2*pi/3  SampleTime=0
  uc : Sin  Amplitude=sqrt(2)*Uf  Frequency=2*pi*fs  Phase=2*pi/3  SampleTime=0
  iRST : Outport  InitialOutput=0
  wires:
  ua/1 -> Mux3/1
  ub/1 -> Mux3/2
  uc/1 -> Mux3/3
  Sum/1 -> Gain/1
  Integrator/1 -> iRST/1, Gain1/1
  Mux3/1 -> Sum/2
  uRST/1 -> Sum/1
  Gain/1 -> Integrator/1
  Gain1/1 -> Sum/3

== system wt_blockset_v3/Grid Models/GRID 2 ==
  iRST : Inport  Port=1  LatchInput=off
  Constant : Constant  Orientation=left  Value=[0 0 0]
  Enabled and Triggered Subsystem : Subsystem  TreatAsAtomicUnit=on
  Gain1 : Gain  Gain=L  SaturateOnIntegerOverflow=on
  Gain2 : Gain  Gain=R  SaturateOnIntegerOverflow=on
  Hit  Crossing : HitCross  HitCrossingDirection=falling
  Mux : Mux  Inputs=3
  Selector : Selector  Elements=[1]  InputPortWidth=3
  Step : Step  Orientation=left  Time=tsc  SampleTime=0
  Step1 : Step  Time=tsc+td  SampleTime=0
  Sum : Sum  Inputs=+-  SaturateOnIntegerOverflow=on  InputSameDT=on
  Sum1 : Sum  Inputs=|++  SaturateOnIntegerOverflow=on  InputSameDT=on
  Sum4 : Sum  Orientation=left  Inputs=+-  SaturateOnIntegerOverflow=on  InputSameDT=on
  Sum5 : Sum  SaturateOnIntegerOverflow=on  InputSameDT=on
  Switch : Switch  Orientation=left  Threshold=0.5
  coeff : Subsystem  mask{N=1e4}
  short_path : Subsystem  Orientation=left
  ua : Sin  Amplitude=sqrt(2)*V1  Frequency=2*pi*fg  SampleTime=0
  ub : Sin  Amplitude=sqrt(2)*V1  Frequency=2*pi*fg  Phase=-2*pi/3  SampleTime=0
  uc : Sin  Amplitude=sqrt(2)*V1  Frequency=2*pi*fg  Phase=2*pi/3  SampleTime=0
  vRST : Outport  InitialOutput=0
  detect : Outport  Port=2  InitialOutput=0
  wires:
  iRST/1 -> Sum5/1
  Gain2/1 -> Sum1/1
  coeff/1(Out1) -> Gain1/1
  Gain1/1 -> Sum1/2
  Sum/1 -> Switch/1, vRST/1
  Sum1/1 -> Sum/2
  Mux/1 -> Sum/1
  Sum5/1 -> Gain2/1, coeff/1(In1)
  Constant/1 -> Switch/3
  Sum4/1 -> Switch/2, detect/1
  Step/1 -> Sum4/1
  Switch/1 -> short_path/1(In1)
  short_path/1(Out1) -> Selector/1, Sum5/2
  Hit  Crossing/1 -> Enabled and Triggered Subsystem/Trigger
  Step1/1 -> Enabled and Triggered Subsystem/1(In1), Enabled and Triggered Subsystem/Enable
  Enabled and Triggered Subsystem/1(Out1) -> Sum4/2
  Selector/1 -> Hit  Crossing/1
  ua/1 -> Mux/1
  ub/1 -> Mux/2
  uc/1 -> Mux/3

== system wt_blockset_v3/Grid Models/Harmonic Voltage Source ==
  ampl : Inport  Port=1  LatchInput=off
  freq : Inport  Port=2  LatchInput=off
  phase : Inport  Port=3  LatchInput=off
  Gain : Gain  Gain=2*pi  SaturateOnIntegerOverflow=on
  Integrator : Integrator
  Mux1 : Mux  Inputs=3
  Mux2 : Mux  Inputs=2
  Phase A : Subsystem
  Phase B : Subsystem
  Phase C : Subsystem
  Sum1 : Sum  Inputs=|++  SaturateOnIntegerOverflow=on
  v_RSTh : Outport
  gama : Outport  Port=2
  wires:
  freq/1 -> Gain/1
  ampl/1 -> Mux2/1
  Gain/1 -> Integrator/1
  Mux1/1 -> v_RSTh/1
  Phase A/1(v_harm) -> Mux1/1
  Phase B/1(v_harm) -> Mux1/2
  Phase C/1(v_harm) -> Mux1/3
  Mux2/1 -> Phase B/1(Input), Phase A/1(Input), Phase C/1(Input)
  Integrator/1 -> Sum1/1
  Sum1/1 -> Mux2/2
  phase/1 -> Sum1/2
  [gama] -> gama/1

== system wt_blockset_v3/Grid Models/Voltage  source complex ==
  Constant : Constant  Value=sqrt(2)*Uf
  Constant1 : Constant  Value=pi/2
  Magnitude-Angle to Complex : MagnitudeAngleToComplex
  V_c : Outport  InitialOutput=0
  wires:
  Constant1/1 -> Magnitude-Angle to Complex/2
  Constant/1 -> Magnitude-Angle to Complex/1
  Magnitude-Angle to Complex/1 -> V_c/1

== system wt_blockset_v3/Measurements/Discrete PLL ==
  V_ABC : Inport  Port=1  LatchInput=off
  Demux : Demux  Outputs=3
  S-Function : S-Function  FunctionName=dscPLL2  Parameters=Kp Ti Ka limit Vrms fgrid ffilter Ts init_cond
  theta : Outport
  Vrms : Outport  Port=2
  fq_grid : Outport  Port=3
  wires:
  S-Function/1 -> Demux/1
  Demux/1 -> theta/1
  V_ABC/1 -> S-Function/1
  Demux/3 -> fq_grid/1
  Demux/2 -> Vrms/1

== system wt_blockset_v3/Measurements/Moving Average Filter ==
  In : Inport  Port=1  LatchInput=off
  Constant : Constant  Value=init
  Gain : Gain  Gain=1/Tav  SaturateOnIntegerOverflow=on
  Integrator : Integrator
  Sum : Sum  Inputs=|+-  SaturateOnIntegerOverflow=on
  Sum1 : Sum  Inputs=|++  SaturateOnIntegerOverflow=on
  Transport Delay : TransportDelay  DelayTime=Tav  InitialInput=init  BufferSize=6144  TransDelayFeedthrough=on
  Out : Outport
  wires:
  In/1 -> Transport Delay/1, Sum/1
  Transport Delay/1 -> Sum/2
  Sum/1 -> Integrator/1
  Integrator/1 -> Gain/1
  Gain/1 -> Sum1/1
  Constant/1 -> Sum1/2
  Sum1/1 -> Out/1

== system wt_blockset_v3/Measurements/P & Q dq ==
  vdq : Inport  Port=1  LatchInput=off
  idq : Inport  Port=2  LatchInput=off
  Active power : Fcn  Expr=1.5*(u(1)*u(3)+u(2)*u(4))
  Mux : Mux  Inputs=[2 2]
  Reactive power : Fcn  Expr=-1.5*(u(1)*u(4)-u(2)*u(3))
  P : Outport
  Q : Outport  Port=2
  wires:
  Mux/1 -> Active power/1, Reactive power/1
  vdq/1 -> Mux/1
  idq/1 -> Mux/2
  Active power/1 -> P/1
  Reactive power/1 -> Q/1

== system wt_blockset_v3/Measurements/P & Q mono phase ==
  v : Inport  Port=1  LatchInput=off
  i : Inport  Port=2  LatchInput=off
  Gain : Gain  Gain=f  SaturateOnIntegerOverflow=on
  Mux : Mux  Inputs=2
  Product : Product  SaturateOnIntegerOverflow=on  InputSameDT=on
  Product1 : Product  SaturateOnIntegerOverflow=on  InputSameDT=on
  Sum1 : Sum  Inputs=+-  SaturateOnIntegerOverflow=on  InputSameDT=on
  T : TransportDelay  DelayTime=1/f1
  T\4 : TransportDelay  DelayTime=1/f/4
  integ : Integrator
  PQ : Outport  InitialOutput=0
  wires:
  Sum1/1 -> Gain/1
  integ/1 -> T/1, Sum1/1
  T/1 -> Sum1/2
  Mux/1 -> integ/1
  Gain/1 -> PQ/1
  Product1/1 -> Mux/2
  Product/1 -> Mux/1
  T\4/1 -> Product1/1
  v/1 -> T\4/1, Product/1
  i/1 -> Product1/2, Product/2

== system wt_blockset_v3/Measurements/P & Q three phase ==
  vabc : Inport  Port=1  LatchInput=off
  iabc : Inport  Port=2  LatchInput=off
  Gain : Gain  Gain=f  SaturateOnIntegerOverflow=on
  Mux : Mux  Inputs=2
  Product1 : Product  SaturateOnIntegerOverflow=on  InputSameDT=on
  Product2 : Product  SaturateOnIntegerOverflow=on  InputSameDT=on
  Sum : Sum  Inputs=+  SaturateOnIntegerOverflow=on
  Sum1 : Sum  Inputs=+-  SaturateOnIntegerOverflow=on  InputSameDT=on
  Sum2 : Sum  Inputs=+  SaturateOnIntegerOverflow=on
  T : TransportDelay  DelayTime=1/f
  T\4 : TransportDelay  DelayTime=1/f/4
  integ : Integrator
  PQ : Outport  InitialOutput=0
  wires:
  Sum2/1 -> Mux/2
  Sum/1 -> Mux/1
  Sum1/1 -> Gain/1
  integ/1 -> T/1, Sum1/1
  T/1 -> Sum1/2
  Mux/1 -> integ/1
  Gain/1 -> PQ/1
  Product1/1 -> Sum2/1
  Product2/1 -> Sum/1
  T\4/1 -> Product1/1
  vabc/1 -> Product2/1, T\4/1
  iabc/1 -> Product2/2, Product1/2

== system wt_blockset_v3/Measurements/Period ==
  input : Inport  Orientation=down  Port=1  LatchInput=off
  Abs : Abs  SaturateOnIntegerOverflow=on
  Clock : Clock
      settings: Decimation=10
  Gain : Gain  Gain=2  SaturateOnIntegerOverflow=on
  Hit  Crossing : HitCross  Orientation=left  HitCrossingOffset=0.01  HitCrossingDirection=rising
  Hit  Crossing1 : HitCross  HitCrossingOffset=0.01  HitCrossingDirection=falling
  Sample and Hold : Subsystem  mask(Sample and Hold){trig=Rising edge, initCond=0}
      mask prompts: trig "Trigger type:"; initCond "Initial condition:"
      mask help: Sample and hold input signal.
      mask init:
      | switch trig
      | case 1, s='rising';
      | case 2, s='falling';
      | case 3, s='either';
      | end
      | set_param([gcb '/Trigger'],'triggertype',s);
      mask Help: web(dspbhelp);
      mask StyleString: popup(Rising edge|Falling edge|Either edge),edit
      mask Display: disp('S/H')
  Sample and Hold1 : Subsystem  mask(Sample and Hold){trig=Falling edge, initCond=0}
      mask prompts: trig "Trigger type:"; initCond "Initial condition:"
      mask help: Sample and hold input signal.
      mask init:
      | switch trig
      | case 1, s='rising';
      | case 2, s='falling';
      | case 3, s='either';
      | end
      | set_param([gcb '/Trigger'],'triggertype',s);
      mask Help: web(dspbhelp);
      mask StyleString: popup(Rising edge|Falling edge|Either edge),edit
      mask Display: disp('S/H')
  Sum1 : Sum  Inputs=+-  SaturateOnIntegerOverflow=on  InputSameDT=on
  T : Outport
  wires:
  Gain/1 -> T/1
  Abs/1 -> Gain/1
  Hit  Crossing1/1 -> Sample and Hold1/Trigger
  input/1 -> Hit  Crossing1/1, Hit  Crossing/1
  Hit  Crossing/1 -> Sample and Hold/Trigger
  Sum1/1 -> Abs/1
  Sample and Hold/1(Out) -> Sum1/1
  Sample and Hold1/1(Out) -> Sum1/2
  Clock/1 -> Sample and Hold1/1(In), Sample and Hold/1(In)

== system wt_blockset_v3/Measurements/Phase Locked Loop ==
  v_RST : Inport  Port=1  LatchInput=off
  Integrator : Integrator
  Mux2 : Mux  Inputs=2
  PI anti wind-up2 : Subsystem  mask{K=Kp, Ti=Ti, ka=10, maxim=100, init_cond=0}
      mask prompts: K "Proportional Constant"; Ti "Integrate constant"; maxim "Limits"; init_cond "initial"
  Product : Product  SaturateOnIntegerOverflow=on
  Product1 : Product  SaturateOnIntegerOverflow=on
  Sum : Sum  Inputs=-+  SaturateOnIntegerOverflow=on
  Sum1 : Sum  Inputs=|++  SaturateOnIntegerOverflow=on
  Trigonometric Function : Trigonometry
  Trigonometric Function1 : Trigonometry  Operator=cos
  base freq : Constant  Orientation=up  Value=2*pi*50
  cos(gama) : Fcn  Expr=u(2)/sqrt(u(1)^2+u(2)^2)
  sin(gama) : Fcn  Expr=u(1)/sqrt(u(1)^2+u(2)^2)
  vx : Fcn  Expr=2/3*u(1)-(u(2)+u(3))/3
  vy : Fcn  Expr=-(u(2)-u(3))/sqrt(3)
  theta : Outport  InitialOutput=0
  wires:
  sin(gama)/1 -> Product1/1
  Product/1 -> Sum/1
  Product1/1 -> Sum/2
  Sum/1 -> PI anti wind-up2/1(ref)
  PI anti wind-up2/1(out) -> Sum1/1
  Sum1/1 -> Integrator/1
  Trigonometric Function/1 -> Product/1
  Trigonometric Function1/1 -> Product1/2
  base freq/1 -> Sum1/2
  Integrator/1 -> Trigonometric Function/1, theta/1, Trigonometric Function1/1
  v_RST/1 -> vx/1, vy/1
  cos(gama)/1 -> Product/2
  vy/1 -> Mux2/2
  vx/1 -> Mux2/1
  Mux2/1 -> cos(gama)/1, sin(gama)/1

== system wt_blockset_v3/Measurements/S complex ==
  u_c : Inport  Port=1  LatchInput=off
  i_c : Inport  Port=2  LatchInput=off
  Gain : Gain  Gain=1.5  SaturateOnIntegerOverflow=on
  Math Function2 : Math  Operator=conj  SaturateOnIntegerOverflow=on
  Product : Product  SaturateOnIntegerOverflow=on  InputSameDT=on
  S_c : Outport
  wires:
  u_c/1 -> Product/1
  i_c/1 -> Math Function2/1
  Product/1 -> Gain/1
  Gain/1 -> S_c/1
  Math Function2/1 -> Product/2

== system wt_blockset_v3/Measurements/average wind ==
  w : Inport  Port=1  LatchInput=off
  Discrete Pulse Generator1 : DiscretePulseGenerator  Period=N_samples  SampleTime=T_sample
  Mean : S-Function  DialogController=dspDDGCreate  DialogControllerArgs=DataTag0  FunctionName=sdspstatfcns  Parameters=fcn,run,reset,0,0,0,dtInfo.accumMode,dtInfo.accumWordLength,dtInfo.accumFracLength,dtInfo.outputMode,dtInfo.outputWordLength,dtInfo.outputFracLength,dtInfo.roundingMode,dtInfo.overflowMode  mask(Mean){run=on, reset_popup=Non-zero sample, additionalParams=off, allowOverrides=on, outputMode=Same as accumulator, outputWordLength=32, outputFracLength=30, accumMode=Same as input, accumWordLength=32, accumFracLength=30, roundingMode=Floor, overflowMode=off, LockScale=off}
      mask prompts: run "Running mean"; reset_popup "Reset port"; additionalParams "--------------- Show additional parameters ---------------"; allowOverrides "Allow overrides from DSP Attributes blocks"; outputMode "Fixed-point output attributes:"; outputWordLength "Output word length:"; outputFracLength "Output fraction length:"; accumMode "Fixed-point accumulator attributes"; accumWordLength "Accumulator word length:"; accumFracLength "Accumulator fraction length:"; roundingMode "Round integer calculations toward:"; overflowMode "Saturate on integer overflow"; LockScale "Lock scaling"
      mask help: Mean of the vector elements. If "Running mean" is selected, the block returns the mean of the input elements over time.
      mask init:
      | [s,x,y] = dspblkmean2('icon');
      | reset=reset_popup-1;
      | fcn=3;
      | dtInfo = dspblkmean2('init');
      settings: CopyFcn=dspfixptcopycallback
      mask Help: web(dspbhelp);
      mask StyleString: checkbox,popup(None|Rising edge|Falling edge|Either edge|Non-zero sample),checkbox,checkbox,popup(Same as accumulator|Same as input|Binary point scaling|Slope and bias scaling|User-defined),edit,edit,popup(Same as input|Binary point scaling|Slope and bias scaling|User-defined),edit,edit,popup(Floor|Nearest),checkbox,checkbox
      mask Display:
      | plot(x,y);
      | port_label('input',s.i1,s.i1s);
      | port_label('input',s.i2,s.i2s);
  Zero-Order Hold : ZeroOrderHold  SampleTime=T_sample
  w_avg : Outport
  wires:
  Mean/1 -> w_avg/1
  w/1 -> Zero-Order Hold/1
  Zero-Order Hold/1 -> Mean/1
  Discrete Pulse Generator1/1 -> Mean/2

== system wt_blockset_v3/Measurements/power spectra ==
  Input : Inport  Port=1  LatchInput=off
  Spectrum Scope : dspsnks4/Spectrum Scope  ScopeProperties=on  Domain=Frequency  HorizSpan=1  UseBuffer=on  BufferSize=1024  Overlap=32  inpFftLenInherit=on  FFTlength=1024  numAvg=3  DisplayProperties=off  AxisGrid=on  Memory=off  FrameNumber=on  AxisLegend=off  AxisZoom=off  OpenScopeAtSimStart=on  OpenScopeImmediately=off  FigPos=get(0,'defaultfigureposition')  AxisProperties=off  XUnits=Hertz  XRange=[0...Fs/2]  InheritXIncr=off  XIncr=0.05  XLabel=Samples  YUnits=dB  YLabel=Magnitude, dB  LineProperties=off  LineColors=[1 0 0]
      settings: YMin=-80  YMax=80
  Zero-Order Hold : ZeroOrderHold  SampleTime=t_sample
  wires:
  Input/1 -> Zero-Order Hold/1
  Zero-Order Hold/1 -> Spectrum Scope/1

== system wt_blockset_v3/Mechanical Components/One-mass model ==
  Tload : Inport  Port=1  LatchInput=off
  Te : Inport  Port=2  LatchInput=off
  Fcn : Fcn  Expr=(pi*50-u(1))/pi/50
  Gain1 : Gain  Gain=1/J  SaturateOnIntegerOverflow=on
  Integrator : Integrator
  Sum : Sum  Inputs=+-  SaturateOnIntegerOverflow=on  InputSameDT=on
  omgr : Outport  InitialOutput=0
  slip : Outport  Port=2  InitialOutput=0
  wires:
  Fcn/1 -> slip/1
  Gain1/1 -> Integrator/1
  Sum/1 -> Gain1/1
  Tload/1 -> Sum/2
  Te/1 -> Sum/1
  Integrator/1 -> Fcn/1, omgr/1

== system wt_blockset_v3/Mechanical Components/One-mass model with gear-box ==
  T_wt : Inport  Port=1  LatchInput=off
  T_em : Inport  Port=2  LatchInput=off
  Gain1 : Gain  Gain=1/J  SaturateOnIntegerOverflow=on
  Gain2 : Gain  Gain=K  SaturateOnIntegerOverflow=on
  Gain3 : Gain  Gain=K  SaturateOnIntegerOverflow=on
  Integrator : Integrator  InitialCondition=init_speed  UpperSaturationLimit=0.95*2*pi*60  LowerSaturationLimit=0
  Sum : Sum  Inputs=+-  SaturateOnIntegerOverflow=on  InputSameDT=on
  omg_wt : Outport  InitialOutput=0
  omg_em : Outport  Port=2  InitialOutput=0
  wires:
  Gain1/1 -> Integrator/1
  Sum/1 -> Gain1/1
  T_em/1 -> Gain3/1
  T_wt/1 -> Sum/1
  Integrator/1 -> omg_wt/1, Gain2/1
  Gain2/1 -> omg_em/1
  Gain3/1 -> Sum/2

== system wt_blockset_v3/Mechanical Components/Two-mass model ==
  T_wt : Inport  Port=1  LatchInput=off
  T_em : Inport  Port=2  LatchInput=off
  Integrator : Integrator  InitialCondition=init(1)
  Integrator1 : Integrator
  Integrator2 : Integrator  InitialCondition=init(2)
  Integrator3 : Integrator
  Mux : Mux  Inputs=6
  domg_em/dt : Fcn  Expr=(-Dshaft*u(1)-Kshaft*u(2)+Dshaft*u(3)*Kgear+Kshaft*Kgear*u(4)+(Kgear^2)*u(6))/(Jem*Kgear^2)
  domg_wt/dt : Fcn  Expr=(Dshaft*u(1)/Kgear+Kshaft*u(2)/Kgear-Dshaft*u(3)-Kshaft*u(4)-u(5))/Jwt
  domg_wt/dt1 : Fcn  Expr=Dshaft*(u(1)/Kgear-u(3))+Kshaft*(u(2)/Kgear-u(4))
  omega_gen : Selector  Elements=[1]  InputPortWidth=6
  omega_gen1 : Selector  Elements=[1]  InputPortWidth=6
  omega_turbine : Selector  Elements=[3]  InputPortWidth=6
  omega_turbine1 : Selector  Elements=[3]  InputPortWidth=6
  omg_em : Outport
  T_shaft : Outport  Port=2
  omg_wt : Outport  Port=3
  wires:
  omega_turbine/1 -> omg_wt/1
  omega_gen/1 -> omg_em/1
  domg_wt/dt1/1 -> T_shaft/1
  T_em/1 -> Mux/6
  T_wt/1 -> Mux/5
  omega_turbine1/1 -> Integrator3/1
  domg_wt/dt/1 -> Integrator2/1
  omega_gen1/1 -> Integrator1/1
  domg_em/dt/1 -> Integrator/1
  Mux/1 -> omega_turbine/1, omega_gen/1, domg_wt/dt1/1, omega_turbine1/1, domg_wt/dt/1, omega_gen1/1, domg_em/dt/1
  Integrator3/1 -> Mux/4  "theta_wt"
  Integrator2/1 -> Mux/3  "omg_wt"
  Integrator1/1 -> Mux/2  "theta_em"
  Integrator/1 -> Mux/1  "omg_em"

== system wt_blockset_v3/Mechanical Components/Two-mass model 'C' S-Function ==
  T_wt : Inport  Port=1  LatchInput=off
  T_em : Inport  Port=2  LatchInput=off
  Demux : Demux  Outputs=3
  Mux : Mux  Inputs=2
  S-Function : S-Function  FunctionName=torsional_torque  Parameters=Jem Jwt Kshaft Dshaft Kgear init_cond
  omg_em : Outport
  T_shaft : Outport  Port=2
  omg_wt : Outport  Port=3
  wires:
  Demux/3 -> T_shaft/1
  Demux/1 -> omg_em/1
  Demux/2 -> omg_wt/1
  S-Function/1 -> Demux/1
  T_em/1 -> Mux/2
  T_wt/1 -> Mux/1
  Mux/1 -> S-Function/1
